simulink model "Braking_noABS_V2"  (R2023b)
settings: Solver=VariableStepAuto  StartTime=0.0  StopTime=3  RelTol=1e-3
values from neighbouring files (symbols this model uses):
  A = 2    [Braking_Param.m]
  c1 = 0.86    [Braking_Param.m]
  c2 = 33.82    [Braking_Param.m]
  c3 = 0.36    [Braking_Param.m]
  cw = 0.3    [Braking_Param.m]
  g = 9.81    [Braking_Param.m]
  Jw = 0.8    [Braking_Param.m]
  m = 1500    [Braking_Param.m]
  Mb = 5350    [Braking_Param.m]
  p = 1.2    [Braking_Param.m]
  rw = 0.3    [Braking_Param.m]
  v0 = 100/3.6    (= 27.7777777778)    [Braking_Param.m]
settings Model: Creator=34266  LastModifiedBy=BeanieBabyJ

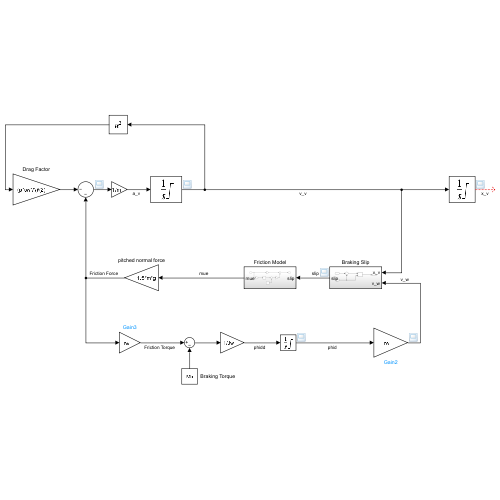
[thumbnail: Simulink's stored preview of the top-level diagram]
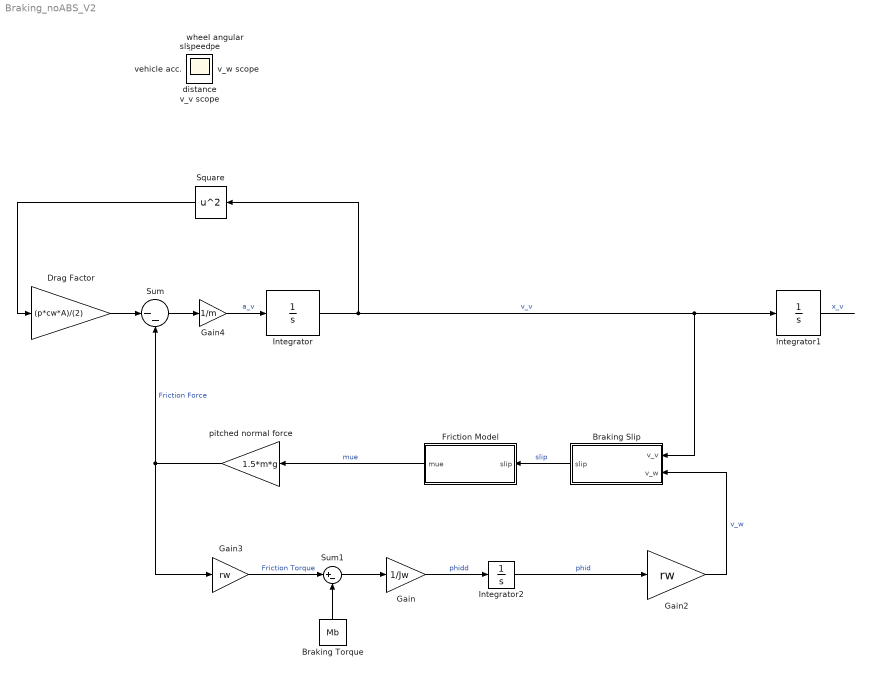
== system Braking_noABS_V2 ==
  Braking Slip : Subsystem
  Braking Torque : Constant  Value=Mb
  Drag Factor : Gain  Gain=(p*cw*A)/(2)
  Friction Model : Subsystem
  Gain : Gain  Gain=1/Jw
  Gain2 : Gain  Gain=rw
  Gain3 : Gain  Gain=rw
  Gain4 : Gain  Gain=1/m
  Integrator : Integrator  InitialCondition=v0  LimitOutput=on  LowerSaturationLimit=0
  Integrator1 : Integrator  LimitOutput=on  LowerSaturationLimit=0
  Integrator2 : Integrator  InitialCondition=v0/rw  LimitOutput=on  LowerSaturationLimit=0
  Square : Math  Operator=square
  Sum : Sum  Inputs=|--
  Sum1 : Sum  Inputs=|+-
  pitched normal force : Gain  Gain=1.5*m*g
  distance : Scope
  slip scope : Scope
  v_v scope : Scope
  v_w scope : Scope
  vehicle acc. : Scope
  wheel angular speed : Scope
  wires:
  Braking Slip/1(slip) -> Friction Model/1(slip)  "slip"
  Integrator/1 -> Square/1, Braking Slip/1(v_v), Integrator1/1  "v_v"
  Sum/1 -> Gain4/1
  pitched normal force/1 -> Sum/2, Gain3/1  "Friction Force"
  Friction Model/1(mue) -> pitched normal force/1  "mue"
  Drag Factor/1 -> Sum/1
  Square/1 -> Drag Factor/1
  Braking Torque/1 -> Sum1/2
  Gain3/1 -> Sum1/1  "Friction Torque"
  Integrator2/1 -> Gain2/1  "phid"
  Gain2/1 -> Braking Slip/2(v_w)  "v_w"
  Integrator1/1 -> ?  "x_v"
  Sum1/1 -> Gain/1
  Gain/1 -> Integrator2/1  "phidd"
  Gain4/1 -> Integrator/1  "a_v"

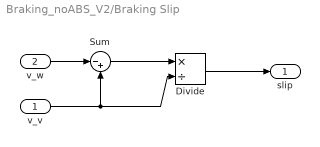
== system Braking_noABS_V2/Braking Slip ==
  v_v : Inport
  v_w : Inport  Port=2
  Divide : Product  Inputs=*/
  Sum : Sum  Inputs=|-+
  slip : Outport
  wires:
  Sum/1 -> Divide/1
  v_v/1 -> Sum/2, Divide/2
  v_w/1 -> Sum/1
  Divide/1 -> slip/1

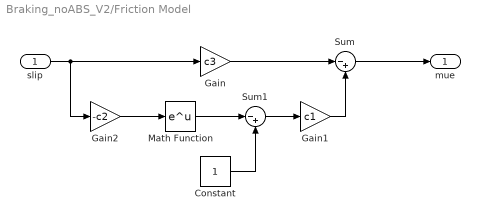
== system Braking_noABS_V2/Friction Model ==
  slip : Inport
  Constant : Constant
  Gain : Gain  Gain=c3
  Gain1 : Gain  Gain=c1
  Gain2 : Gain  Gain=-c2
  Math Function : Math
  Sum : Sum  Inputs=|-+
  Sum1 : Sum  Inputs=|-+
  mue : Outport
  wires:
  Sum1/1 -> Gain1/1
  slip/1 -> Gain/1, Gain2/1
  Gain2/1 -> Math Function/1
  Math Function/1 -> Sum1/1
  Constant/1 -> Sum1/2
  Gain1/1 -> Sum/2
  Gain/1 -> Sum/1
  Sum/1 -> mue/1
